simulink model "AD_9S12"  (Simulink 10.0)
settings: Solver=ode1  StartTime=0.0  StopTime=inf  FixedStep=0.002  RelTol=1e-3
settings Model: Creator=Admin  LastModifiedBy=bhisma  SimulationMode=external
settings ConfigSet: Description=rtmc9s12target_R2009b
settings DataIOCC: LimitDataPoints=on  SignalLoggingSaveFormat=ModelDataLogs  SaveOutput=off  SaveTime=off  SignalLoggingName=sigsOut
settings OptimizationCC: ExpressionDepthLimit=2147483647  InitFltsAndDblsToZero=on  LifeSpan=1  EfficientTunableParamExpr=on
settings DebuggingCC: SaveWithParameterizedLinksMsg=none  SignalResolutionControl=TryResolveAllWithWarning  MultiTaskDSMMsg=warning  MultiTaskCondExecSysMsg=none  FcnCallInpInsideContextMsg=warning  StateNameClashWarn=warning
settings HardwareCC: ProdBitPerInt=16  ProdBitPerPointer=16  ProdBitPerSizeT=16  ProdBitPerPtrDiffT=16  ProdEndianess=BigEndian  ProdWordSize=16  ProdHWDeviceType=Motorola HC12  TargetHWDeviceType=32-bit Generic
settings SFSimCC: MATLABDynamicMemAlloc=off
settings RTWCC: Description=rtmc9s12-Target for Metrowerks CodeWarrior  SystemTargetFile=mc9s12.tlc  GenerateMakefile=off  TemplateMakefile=mc9s12.tmf
settings CodeAppCC: CustomSymbolStrType=$N$R$M  InternalIdentifier=Classic
settings STFCustomTargetCC: TargetFcnLib=ansi_tfl_tmw.mat  ModelReferenceCompliant=off  IncludeMdlTerminateFcn=off  ERTCustomFileBanners=on  SupportNonInlinedSFcns=off  RemoveResetFunc=on  MATLABClassNameForMDSCustomization=Simulink.SoftwareTarget.ERTCustomization  CPPClassGenCompliant=on  SystemTargetFile=mc9s12.tlc
settings ERTTargetCC: TargetFcnLib=ansi_tfl_tmw.mat  MultiwordLength=2048  ModelReferenceCompliant=off  ParMdlRefBuildCompliant=off  CompOptLevelCompliant=off  ConcurrentExecutionCompliant=off  IncludeMdlTerminateFcn=off  CombineOutputUpdateFcns=off  SupportContinuousTime=on  ModelStepFunctionPrototypeControlCompliant=off  GRTInterface=on  UseToolchainInfoCompliant=off  ExtMode=on  ExtModeMexFile=ext_serial_mc9s12_comm  ExtModeMexArgs=1,2,115200  ERTCustomFileTemplate=mc9s12_file_process.tlc  ConvertIfToSwitch=off  SuppressUnreachableDefaultCases=off
settings CustomProperty: DataType=RTWOptions_EnumType_C__Users_fw__SVN_rtmc9s12-target_trunk_rtmc9s12_CW_R2009b_bin_mc9s12_1mc9s12_TargetBoard  Value=Dragon12Plus
settings EnumStrPairs: String=Dragon12
settings ConfigComp: CovExternalEMLEnable=off

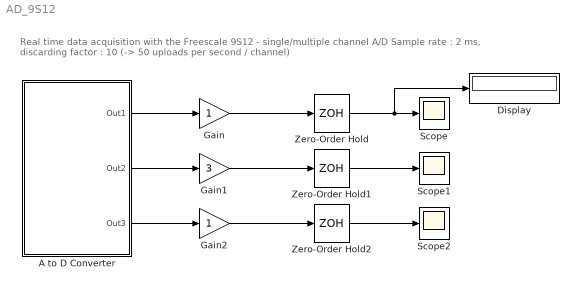
== system AD_9S12 ==
  note: Real time data acquisition with the Freescale 9S12 - single/multiple channel A/D
      | Sample rate : 2 ms, discarding factor : 10 (-> 50 uploads per second / channel)
  A to D Converter : Subsystem  Tag=mcTarget_adc  mask{bank=0, channels=5 - 7, use10bits=10 bits, normalize=max. output:  5, sampletime=0.002}
      mask prompts: bank "ADC bank"; channels "Channels ( 0 - 7 )"; use10bits "ADC resolution"; normalize "Normalization"; sampletime "Sample time"
      mask init:
      | [channelsStr, firstChannel, numChannels] = mbc_adcinput(channels);
      mask Help: web('adc_sfcn_9S12.html');
      mask TypeOptions bank: 0 | 1
      mask TypeOptions use10bits: 10 bits | 8 bits
      mask TypeOptions normalize: raw values | max. output:  1 | max. output:  5
      mask Display: disp(['A to D Converter\n' channelsStr])
  Display : Display
  Gain : Gain  SaturateOnIntegerOverflow=on  OutDataTypeStr=Inherit: Same as input  ParamDataTypeStr=Inherit: Same as input
  Gain1 : Gain  Gain=3  SaturateOnIntegerOverflow=on  OutDataTypeStr=Inherit: Same as input  ParamDataTypeStr=Inherit: Same as input
  Gain2 : Gain  SaturateOnIntegerOverflow=on  OutDataTypeStr=Inherit: Same as input  ParamDataTypeStr=Inherit: Same as input
  Scope : Scope
  Scope1 : Scope
  Scope2 : Scope
  Zero-Order Hold : ZeroOrderHold  SampleTime=0.02
  Zero-Order Hold1 : ZeroOrderHold  SampleTime=0.02
  Zero-Order Hold2 : ZeroOrderHold  SampleTime=0.02
  wires:
  A to D Converter/1(Out1) -> Gain/1
  Zero-Order Hold/1 -> Scope/1, Display/1
  Gain/1 -> Zero-Order Hold/1
  A to D Converter/2(Out2) -> Gain1/1
  Zero-Order Hold1/1 -> Scope1/1
  Gain1/1 -> Zero-Order Hold1/1
  Zero-Order Hold2/1 -> Scope2/1
  Gain2/1 -> Zero-Order Hold2/1
  A to D Converter/3(Out3) -> Gain2/1

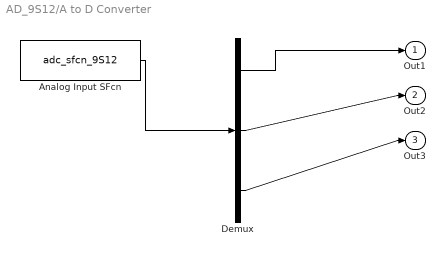
== system AD_9S12/A to D Converter ==
  Analog Input SFcn : S-Function  Tag=mcTarget_adc  FunctionName=adc_sfcn_9S12  Parameters=bank-1, firstChannel, numChannels, use10bits-1, normalize, sampletime  SFunctionDeploymentMode=off  EnableBusSupport=off
  Demux : Demux  Outputs=3
  Out1 : Outport
  Out2 : Outport  Port=2
  Out3 : Outport  Port=3
  wires:
  Analog Input SFcn/1 -> Demux/1
  Demux/1 -> Out1/1
  Demux/2 -> Out2/1
  Demux/3 -> Out3/1
